simulink model "CoVMD"  (R2018a)
settings: configuration reference "cs_ert" (kept outside this file)
settings Model: DataDictionary=CoVMD.sldd  Creator=zhoutinglin  LastModifiedBy=zhoutinglin

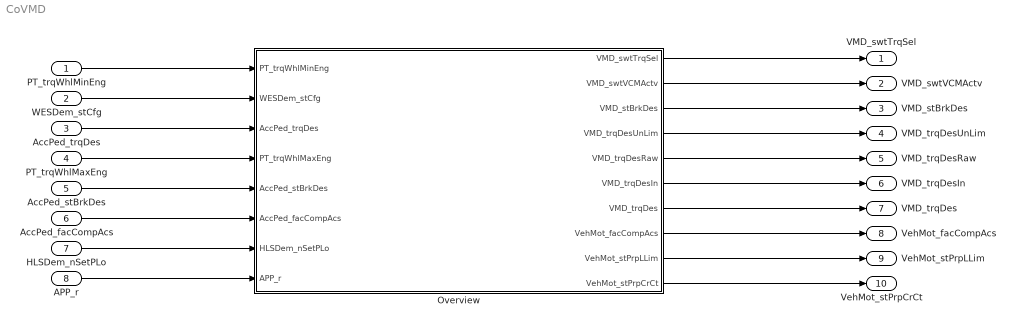
== system CoVMD ==
  PT_trqWhlMinEng : Inport
  WESDem_stCfg : Inport  Port=2
  AccPed_trqDes : Inport  Port=3
  PT_trqWhlMaxEng : Inport  Port=4
  AccPed_stBrkDes : Inport  Port=5
  AccPed_facCompAcs : Inport  Port=6
  HLSDem_nSetPLo : Inport  Port=7
  APP_r : Inport  Port=8
  Overview : Subsystem
  VMD_swtTrqSel : Outport
  VMD_swtVCMActv : Outport  Port=2
  VMD_stBrkDes : Outport  Port=3
  VMD_trqDesUnLim : Outport  Port=4
  VMD_trqDesRaw : Outport  Port=5
  VMD_trqDesIn : Outport  Port=6
  VMD_trqDes : Outport  Port=7
  VehMot_facCompAcs : Outport  Port=8
  VehMot_stPrpLLim : Outport  Port=9
  VehMot_stPrpCrCt : Outport  Port=10
  wires:
  PT_trqWhlMinEng/1 -> Overview/1(PT_trqWhlMinEng)
  WESDem_stCfg/1 -> Overview/2(WESDem_stCfg)
  AccPed_trqDes/1 -> Overview/3(AccPed_trqDes)
  PT_trqWhlMaxEng/1 -> Overview/4(PT_trqWhlMaxEng)
  AccPed_stBrkDes/1 -> Overview/5(AccPed_stBrkDes)
  AccPed_facCompAcs/1 -> Overview/6(AccPed_facCompAcs)
  HLSDem_nSetPLo/1 -> Overview/7(HLSDem_nSetPLo)
  APP_r/1 -> Overview/8(APP_r)
  Overview/1(VMD_swtTrqSel) -> VMD_swtTrqSel/1
  Overview/2(VMD_swtVCMActv) -> VMD_swtVCMActv/1
  Overview/3(VMD_stBrkDes) -> VMD_stBrkDes/1
  Overview/4(VMD_trqDesUnLim) -> VMD_trqDesUnLim/1
  Overview/5(VMD_trqDesRaw) -> VMD_trqDesRaw/1
  Overview/6(VMD_trqDesIn) -> VMD_trqDesIn/1
  Overview/7(VMD_trqDes) -> VMD_trqDes/1
  Overview/8(VehMot_facCompAcs) -> VehMot_facCompAcs/1
  Overview/9(VehMot_stPrpLLim) -> VehMot_stPrpLLim/1
  Overview/10(VehMot_stPrpCrCt) -> VehMot_stPrpCrCt/1

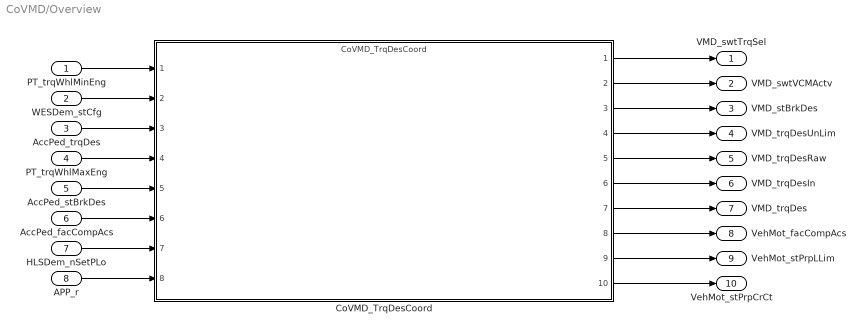
== system CoVMD/Overview ==
  PT_trqWhlMinEng : Inport
  WESDem_stCfg : Inport  Port=2
  AccPed_trqDes : Inport  Port=3
  PT_trqWhlMaxEng : Inport  Port=4
  AccPed_stBrkDes : Inport  Port=5
  AccPed_facCompAcs : Inport  Port=6
  HLSDem_nSetPLo : Inport  Port=7
  APP_r : Inport  Port=8
  CoVMD_TrqDesCoord : ModelReference  ModelNameDialog=CoVMD_TrqDesCoord  SimulationMode=Normal  ModelReferenceVersion=1.54
  VMD_swtTrqSel : Outport
  VMD_swtVCMActv : Outport  Port=2
  VMD_stBrkDes : Outport  Port=3
  VMD_trqDesUnLim : Outport  Port=4
  VMD_trqDesRaw : Outport  Port=5
  VMD_trqDesIn : Outport  Port=6
  VMD_trqDes : Outport  Port=7
  VehMot_facCompAcs : Outport  Port=8
  VehMot_stPrpLLim : Outport  Port=9
  VehMot_stPrpCrCt : Outport  Port=10
  wires:
  PT_trqWhlMinEng/1 -> CoVMD_TrqDesCoord/1
  WESDem_stCfg/1 -> CoVMD_TrqDesCoord/2
  AccPed_trqDes/1 -> CoVMD_TrqDesCoord/3
  PT_trqWhlMaxEng/1 -> CoVMD_TrqDesCoord/4
  AccPed_stBrkDes/1 -> CoVMD_TrqDesCoord/5
  AccPed_facCompAcs/1 -> CoVMD_TrqDesCoord/6
  HLSDem_nSetPLo/1 -> CoVMD_TrqDesCoord/7
  APP_r/1 -> CoVMD_TrqDesCoord/8
  CoVMD_TrqDesCoord/1 -> VMD_swtTrqSel/1
  CoVMD_TrqDesCoord/2 -> VMD_swtVCMActv/1
  CoVMD_TrqDesCoord/3 -> VMD_stBrkDes/1
  CoVMD_TrqDesCoord/4 -> VMD_trqDesUnLim/1
  CoVMD_TrqDesCoord/5 -> VMD_trqDesRaw/1
  CoVMD_TrqDesCoord/6 -> VMD_trqDesIn/1
  CoVMD_TrqDesCoord/7 -> VMD_trqDes/1
  CoVMD_TrqDesCoord/8 -> VehMot_facCompAcs/1
  CoVMD_TrqDesCoord/9 -> VehMot_stPrpLLim/1
  CoVMD_TrqDesCoord/10 -> VehMot_stPrpCrCt/1
